simulink model "modelo_LTI_controlador_parcial"  (R2020a)
settings: Solver=VariableStepAuto  StartTime=0.0  StopTime=10.0  RelTol=1e-3
model workspace: external: MATLAB File D:\Ferran\Facultad\UNCuyo\Meca\Automática y Máquinas Eléctricas\Proyecto final\matlab2\parametros_y_especs\parametros_y_especif.m (data not in the file)
undefined symbols (not defined in the file): alpha_Cu, beq, Cts, Jeq, L_ls, lambda_m, Ld, Lq, Pp, r, Rref, Rts_amb, Tref
settings Model: Creator=Ferran  LastModifiedBy=Ferran

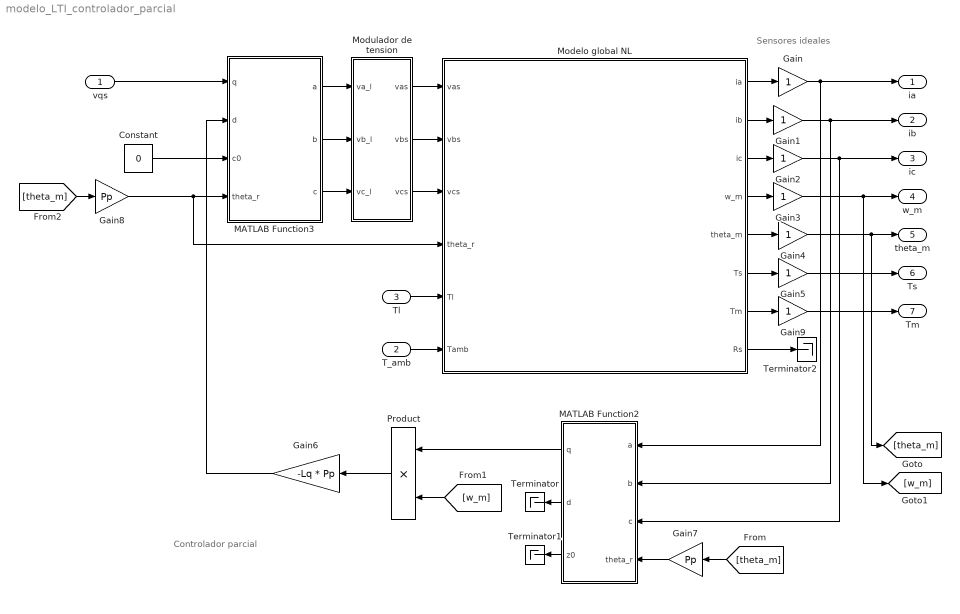
== system modelo_LTI_controlador_parcial ==
  note: Controlador parcial
  note: Sensores ideales
  vqs : Inport
  T_amb : Inport  Port=2
  Tl : Inport  Port=3
  Constant : Constant  Value=0
  Gain{,1..5,9} (7 alike) : Gain
  Gain6 : Gain  Gain=-Lq * Pp
  Gain7 : Gain  Gain=Pp
  Gain8 : Gain  Gain=Pp
  MATLAB Function2 : MATLAB Function  TreatAsAtomicUnit=on
  MATLAB Function3 : MATLAB Function  TreatAsAtomicUnit=on
  Modelo global NL : Subsystem
  Modulador de tension : Subsystem
  Product : Product
  Terminator : Terminator
  Terminator1 : Terminator
  Terminator2 : Terminator
  ia : Outport
  ib : Outport  Port=2
  ic : Outport  Port=3
  w_m : Outport  Port=4
  theta_m : Outport  Port=5
  Ts : Outport  Port=6
  Tm : Outport  Port=7
  wires:
  Modelo global NL/1(ia) -> Gain/1
  Modelo global NL/2(ib) -> Gain1/1
  Modelo global NL/3(ic) -> Gain2/1
  Modelo global NL/4(w_m) -> Gain3/1
  Modelo global NL/5(theta_m) -> Gain4/1
  Modelo global NL/6(Ts) -> Gain5/1
  Gain/1 -> MATLAB Function2/1(a), ia/1
  Gain1/1 -> MATLAB Function2/2(b), ib/1
  Gain2/1 -> MATLAB Function2/3(c), ic/1
  Modulador de tension/1(vas) -> Modelo global NL/1(vas)
  Modulador de tension/2(vbs) -> Modelo global NL/2(vbs)
  Modulador de tension/3(vcs) -> Modelo global NL/3(vcs)
  MATLAB Function3/1(a) -> Modulador de tension/1(va_l)
  MATLAB Function3/2(b) -> Modulador de tension/2(vb_l)
  MATLAB Function3/3(c) -> Modulador de tension/3(vc_l)
  Gain3/1 -> w_m/1, [w_m]
  Gain4/1 -> [theta_m], theta_m/1
  Gain5/1 -> Ts/1
  Constant/1 -> MATLAB Function3/3(c0)
  MATLAB Function2/2(d) -> Terminator/1
  MATLAB Function2/3(z0) -> Terminator1/1
  MATLAB Function2/1(q) -> Product/1
  Product/1 -> Gain6/1
  Gain6/1 -> MATLAB Function3/2(d)
  [theta_m] -> Gain7/1
  Gain7/1 -> MATLAB Function2/4(theta_r)
  [w_m] -> Product/2
  [theta_m] -> Gain8/1
  Gain8/1 -> MATLAB Function3/4(theta_r), Modelo global NL/4(theta_r)
  vqs/1 -> MATLAB Function3/1(q)
  T_amb/1 -> Modelo global NL/6(Tamb)
  Tl/1 -> Modelo global NL/5(Tl)
  Modelo global NL/7(Tm) -> Gain9/1
  Gain9/1 -> Tm/1
  Modelo global NL/8(Rs) -> Terminator2/1

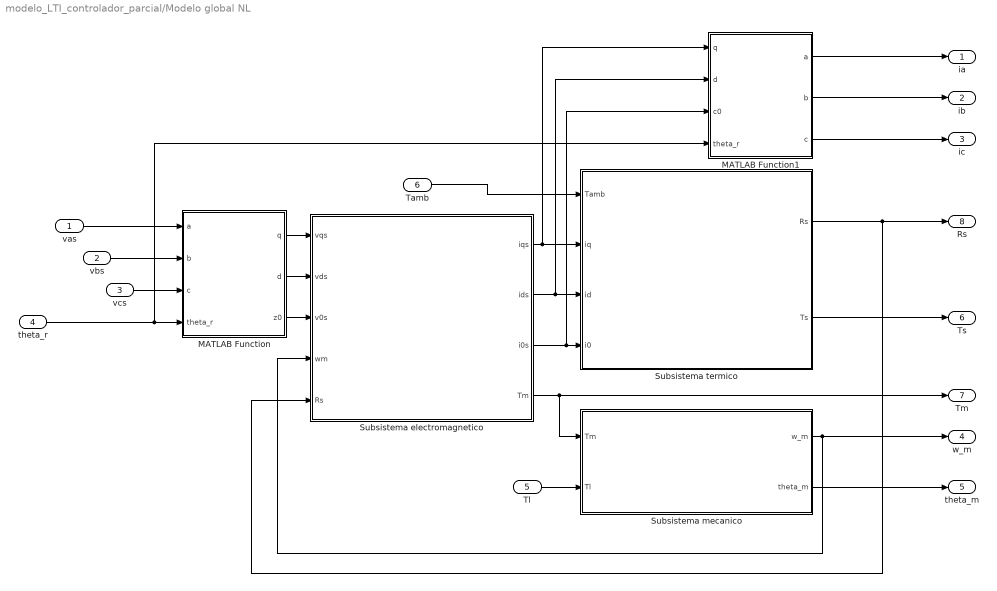
== system modelo_LTI_controlador_parcial/Modelo global NL ==
  vas : Inport
  vbs : Inport  Port=2
  vcs : Inport  Port=3
  theta_r : Inport  Port=4
  Tl : Inport  Port=5
  Tamb : Inport  Port=6
  MATLAB Function : MATLAB Function  TreatAsAtomicUnit=on
  MATLAB Function1 : MATLAB Function  TreatAsAtomicUnit=on
  Subsistema electromagnetico : Subsystem
  Subsistema mecanico : Subsystem
  Subsistema termico : Subsystem
  ia : Outport
  ib : Outport  Port=2
  ic : Outport  Port=3
  w_m : Outport  Port=4
  theta_m : Outport  Port=5
  Ts : Outport  Port=6
  Tm : Outport  Port=7
  Rs : Outport  Port=8
  wires:
  MATLAB Function1/3(c) -> ic/1
  MATLAB Function1/2(b) -> ib/1
  Subsistema electromagnetico/4(Tm) -> Tm/1, Subsistema mecanico/1(Tm)
  Subsistema termico/2(Ts) -> Ts/1
  MATLAB Function/1(q) -> Subsistema electromagnetico/1(vqs)
  Subsistema termico/1(Rs) -> Rs/1, Subsistema electromagnetico/5(Rs)
  Subsistema electromagnetico/2(ids) -> MATLAB Function1/2(d), Subsistema termico/3(id)
  Subsistema mecanico/1(w_m) -> w_m/1, Subsistema electromagnetico/4(wm)
  Tamb/1 -> Subsistema termico/1(Tamb)
  Subsistema mecanico/2(theta_m) -> theta_m/1
  MATLAB Function1/1(a) -> ia/1
  Subsistema electromagnetico/1(iqs) -> MATLAB Function1/1(q), Subsistema termico/2(iq)
  vas/1 -> MATLAB Function/1(a)
  Subsistema electromagnetico/3(i0s) -> MATLAB Function1/3(c0), Subsistema termico/4(i0)
  vcs/1 -> MATLAB Function/3(c)
  Tl/1 -> Subsistema mecanico/2(Tl)
  vbs/1 -> MATLAB Function/2(b)
  MATLAB Function/2(d) -> Subsistema electromagnetico/2(vds)
  MATLAB Function/3(z0) -> Subsistema electromagnetico/3(v0s)
  theta_r/1 -> MATLAB Function1/4(theta_r), MATLAB Function/4(theta_r)

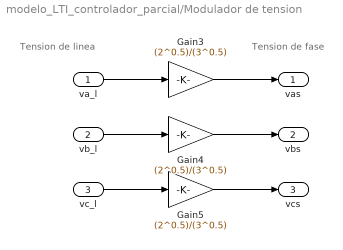
== system modelo_LTI_controlador_parcial/Modulador de tension ==
  note: Tension de fase
  note: Tension de linea
  va_l : Inport
  vb_l : Inport  Port=2
  vc_l : Inport  Port=3
  Gain3 : Gain  Gain=(2^0.5)/(3^0.5)
  Gain4 : Gain  Gain=(2^0.5)/(3^0.5)
  Gain5 : Gain  Gain=(2^0.5)/(3^0.5)
  vas : Outport
  vbs : Outport  Port=2
  vcs : Outport  Port=3
  wires:
  Gain4/1 -> vbs/1
  va_l/1 -> Gain3/1
  Gain5/1 -> vcs/1
  vb_l/1 -> Gain4/1
  vc_l/1 -> Gain5/1
  Gain3/1 -> vas/1

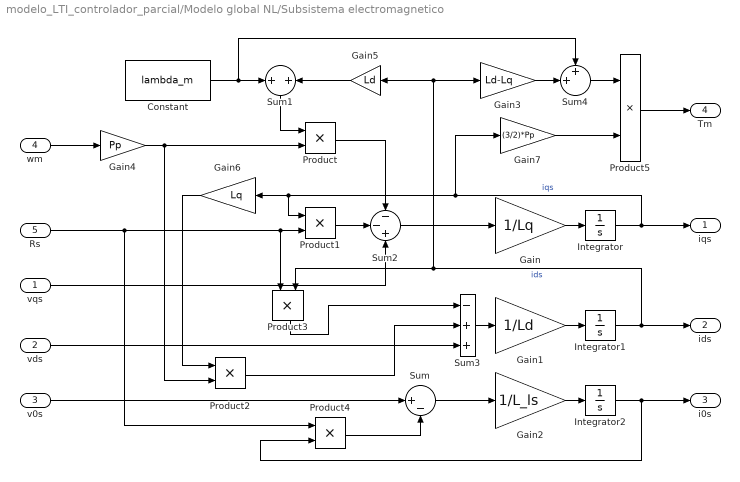
== system modelo_LTI_controlador_parcial/Modelo global NL/Subsistema electromagnetico ==
  vqs : Inport
  vds : Inport  Port=2
  v0s : Inport  Port=3
  wm : Inport  Port=4
  Rs : Inport  Port=5
  Constant : Constant  Value=lambda_m
  Gain : Gain  Gain=1/Lq
  Gain1 : Gain  Gain=1/Ld
  Gain2 : Gain  Gain=1/L_ls
  Gain3 : Gain  Gain=Ld-Lq
  Gain4 : Gain  Gain=Pp
  Gain5 : Gain  Gain=Ld
  Gain6 : Gain  Gain=Lq
  Gain7 : Gain  Gain=(3/2)*Pp
  Integrator : Integrator
  Integrator1 : Integrator
  Integrator2 : Integrator
  Product{,1..5} (6 alike) : Product
  Sum : Sum  Inputs=|+-
  Sum1 : Sum  Inputs=+|+
  Sum2 : Sum  Inputs=--+
  Sum3 : Sum  Inputs=-++
  Sum4 : Sum  Inputs=++|
  iqs : Outport
  ids : Outport  Port=2
  i0s : Outport  Port=3
  Tm : Outport  Port=4
  wires:
  Constant/1 -> Sum1/1, Sum4/1
  Product1/1 -> Sum2/2
  Rs/1 -> Product1/2, Product3/1, Product4/1
  Integrator/1 -> iqs/1, Gain7/1, Gain6/1, Product1/1  "iqs"
  Gain3/1 -> Sum4/2
  Sum/1 -> Gain2/1
  Sum2/1 -> Gain/1
  vqs/1 -> Sum2/3
  Product3/1 -> Sum3/1
  Product4/1 -> Sum/2
  vds/1 -> Sum3/3
  Sum3/1 -> Gain1/1
  Gain6/1 -> Product2/1
  Integrator1/1 -> ids/1, Product3/2, Gain5/1, Gain3/1  "ids"
  Product2/1 -> Sum3/2
  Integrator2/1 -> i0s/1, Product4/2
  wm/1 -> Gain4/1
  Sum1/1 -> Product/1
  Gain5/1 -> Sum1/2
  Product/1 -> Sum2/1
  Gain/1 -> Integrator/1
  v0s/1 -> Sum/1
  Gain2/1 -> Integrator2/1
  Gain1/1 -> Integrator1/1
  Gain7/1 -> Product5/2
  Product5/1 -> Tm/1
  Gain4/1 -> Product/2, Product2/2
  Sum4/1 -> Product5/1

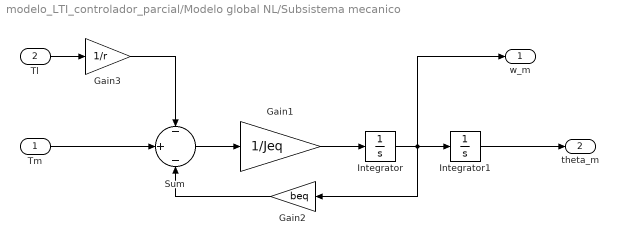
== system modelo_LTI_controlador_parcial/Modelo global NL/Subsistema mecanico ==
  Tm : Inport
  Tl : Inport  Port=2
  Gain1 : Gain  Gain=1/Jeq
  Gain2 : Gain  Gain=beq
  Gain3 : Gain  Gain=1/r
  Integrator : Integrator
  Integrator1 : Integrator
  Sum : Sum  Inputs=-|+|-
  w_m : Outport
  theta_m : Outport  Port=2
  wires:
  Tm/1 -> Sum/2
  Gain3/1 -> Sum/1
  Integrator/1 -> w_m/1, Gain2/1, Integrator1/1
  Integrator1/1 -> theta_m/1
  Gain2/1 -> Sum/3
  Sum/1 -> Gain1/1
  Tl/1 -> Gain3/1
  Gain1/1 -> Integrator/1

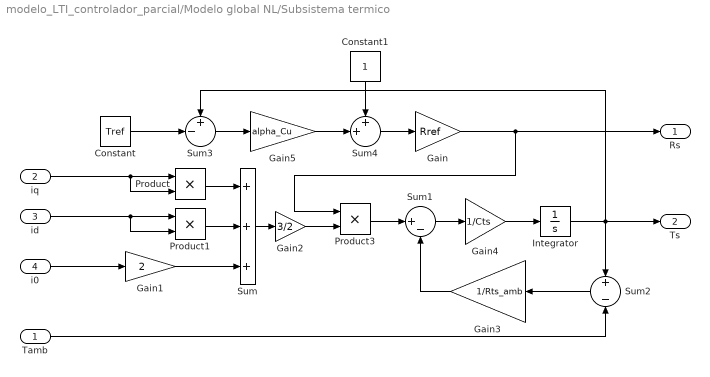
== system modelo_LTI_controlador_parcial/Modelo global NL/Subsistema termico ==
  Tamb : Inport
  iq : Inport  Port=2
  id : Inport  Port=3
  i0 : Inport  Port=4
  Constant : Constant  Value=Tref
  Constant1 : Constant
  Gain : Gain  Gain=Rref
  Gain1 : Gain  Gain=2
  Gain2 : Gain  Gain=3/2
  Gain3 : Gain  Gain=1/Rts_amb
  Gain4 : Gain  Gain=1/Cts
  Gain5 : Gain  Gain=alpha_Cu
  Integrator : Integrator  InitialCondition=20
  Product : Product
  Product1 : Product
  Product3 : Product
  Sum : Sum  Inputs=+++
  Sum1 : Sum  Inputs=|+-
  Sum2 : Sum  Inputs=+-
  Sum3 : Sum  Inputs=+-|
  Sum4 : Sum  Inputs=++|
  Rs : Outport
  Ts : Outport  Port=2
  wires:
  Gain1/1 -> Sum/3
  Constant/1 -> Sum3/2
  iq/1 -> Product/1, Product/2
  Product3/1 -> Sum1/1
  Integrator/1 -> Ts/1, Sum3/1, Sum2/1
  Gain4/1 -> Integrator/1
  id/1 -> Product1/1, Product1/2
  Sum3/1 -> Gain5/1
  Constant1/1 -> Sum4/1
  Sum4/1 -> Gain/1
  Gain3/1 -> Sum1/2
  Tamb/1 -> Sum2/2
  Sum1/1 -> Gain4/1
  Gain/1 -> Rs/1, Product3/1
  Product1/1 -> Sum/2
  i0/1 -> Gain1/1
  Gain2/1 -> Product3/2
  Product/1 -> Sum/1
  Gain5/1 -> Sum4/2
  Sum/1 -> Gain2/1
  Sum2/1 -> Gain3/1

== matlab function modelo_LTI_controlador_parcial/Modelo global NL/MATLAB Function1 ==
  data: q input; a output; d input; c0 input; theta_r input; b output; c output
function [a,b,c] = TPark_inversa(q,d,c0,theta_r)
    fqd0 = [q;d;c0];
    T = [cos(theta_r)               sin(theta_r)            1;
        cos(theta_r - (2*pi)/3)    sin(theta_r - (2*pi)/3) 1;
        cos(theta_r + (2*pi)/3)    sin(theta_r + (2*pi)/3) 1];
    
    fabc = T*fqd0;
    
    a = fabc(1);
    b = fabc(2);
    c = fabc(3);
end

== matlab function modelo_LTI_controlador_parcial/Modelo global NL/MATLAB Function ==
  data: a input; q output; b input; c input; theta_r input; d output; z0 output
function [q,d,z0] = TPark_directa(a,b,c,theta_r)
    fabc = [a;b;c];
    T = (2/3) * ...
        [ cos(theta_r) cos(theta_r - (2*pi)/3) cos(theta_r + (2*pi)/3);
        sin(theta_r) sin(theta_r - (2*pi)/3) sin(theta_r + (2*pi)/3);
        1/2                   1/2                  1/2];
  
  fqd0 = T*fabc;
  q = fqd0(1);
  d = fqd0(2);
  z0 = fqd0(3);
end

== matlab function modelo_LTI_controlador_parcial/MATLAB Function2 ==
  data: a input; q output; b input; c input; theta_r input; d output; z0 output
function [q,d,z0] = TPark_directa(a,b,c,theta_r)
    fabc = [a;b;c];
    T = (2/3) * ...
        [ cos(theta_r) cos(theta_r - (2*pi)/3) cos(theta_r + (2*pi)/3);
        sin(theta_r) sin(theta_r - (2*pi)/3) sin(theta_r + (2*pi)/3);
        1/2                   1/2                  1/2];
  
  fqd0 = T*fabc;
  q = fqd0(1);
  d = fqd0(2);
  z0 = fqd0(3);
end

== matlab function modelo_LTI_controlador_parcial/MATLAB Function3 ==
  data: q input; a output; d input; c0 input; theta_r input; b output; c output
function [a,b,c] = TPark_inversa(q,d,c0,theta_r)
    fqd0 = [q;d;c0];
    T = [cos(theta_r)               sin(theta_r)            1;
        cos(theta_r - (2*pi)/3)    sin(theta_r - (2*pi)/3) 1;
        cos(theta_r + (2*pi)/3)    sin(theta_r + (2*pi)/3) 1];
    
    fabc = T*fqd0;
    
    a = fabc(1);
    b = fabc(2);
    c = fabc(3);
end
